simulink model "RobotPID"  (R2023b)
settings: Solver=ode23t  StartTime=0.0  StopTime=inf  RelTol=1e-3
InitFcn:
  | RPInit
StopFcn:
  | run('OccupancyMap.m');
model workspace (MAT data in the model file):
  mapForSim : object (value not decoded)
  occGrid : robotics.BinaryOccupancyGrid (value not decoded)
values from neighbouring files (symbols this model uses):
  X = X + abs(minX)    [OccupancyMap.m]
  Y = Y + abs(minY)    [OccupancyMap.m]
undefined symbols (not defined in the file or in its folder): FloorSurface, Ref, RobotSurface, Z
libraries: sm_lib x21, RP_Simulator_Components x13, nesl_utility x11, RoboticsPlayground x6, slpidlib x2
(part 2 of 2)

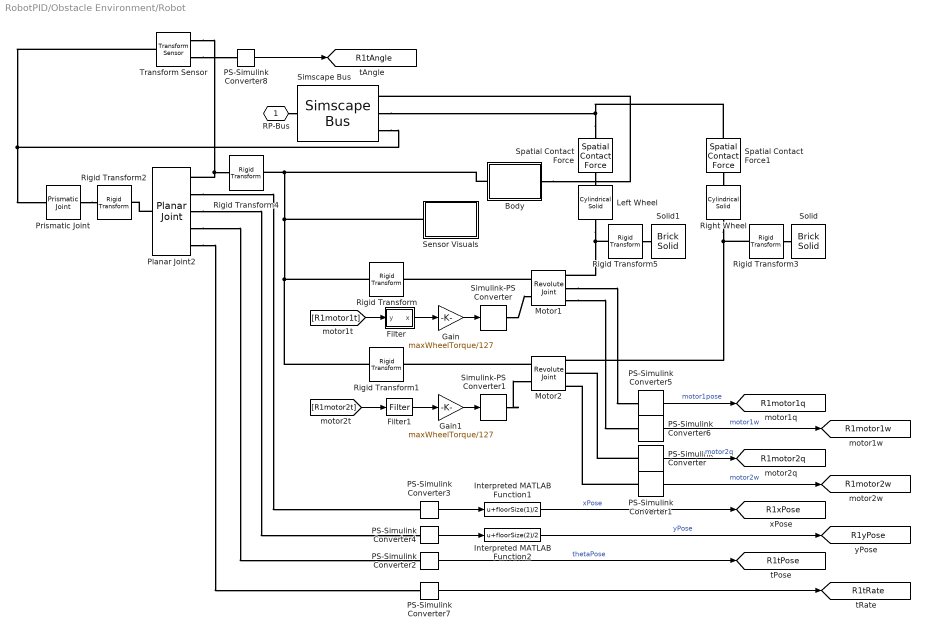
== system RobotPID/Obstacle Environment/Robot ==
  Body : Subsystem
  Filter : Subsystem
  Filter1 : RP_Simulator_Components/Contact Tank Robot/Filter  SystemSampleTime=-1  VariantActivationTime=update diagram  AllowFlexibleInterface=on  Latency=0  AutoFrameSizeCalculation=off
  Gain : Gain  Gain=maxWheelTorque/127
  Gain1 : Gain  Gain=maxWheelTorque/127
  Interpreted MATLAB Function1 : MATLABFcn  MATLABFcn=u+floorSize(1)/2
  Interpreted MATLAB Function2 : MATLABFcn  MATLABFcn=u+floorSize(2)/2
  Left Wheel : sm_lib/Body Elements/Cylindrical Solid  GraphicAmbientColor=[0.15 0.15 0.15 1.0]  BasedOnType=Mass  CenterOfMass=[0 0 0]  CenterOfMassUnits=m  GraphicDiffuseColor=wheelColor  CylinderLength=wheelThickness  CylinderLengthUnits=m  CylinderRadius=wheelRadius  CylinderRadiusUnits=m  Density=1000  DensityUnits=kg/m^3  DoExposeReferenceFrame=on  GraphicEmissiveColor=[0.0 0.0 0.0 1.0]  ExportEntireGeometry=on  SerializedFrames=<Frames/>  MarkerShape=Sphere  MarkerSize=10  GraphicType=FromGeometry  InertiaType=CalculateFromGeometry  Mass=wheelMass  MassUnits=kg  MomentsOfInertia=[1 1 1]  MomentsOfInertiaUnits=kg*m^2  GraphicOpacity=1.0  ProductsOfInertia=[1 1 1]  ProductsOfInertiaUnits=kg*m^2  GraphicShininess=75  GraphicSpecularColor=[0.5 0.5 0.5 1.0]  GraphicVisPropType=SimpleVisualProperties
  Motor1 : sm_lib/Joints/Revolute Joint  JointMode=Normal  SenseConstraintForce=off  SenseConstraintForceX=off  SenseConstraintForceY=off  SenseConstraintForceZ=off  SenseConstraintTorque=off  SenseConstraintTorqueX=off  SenseConstraintTorqueY=off  SenseConstraintTorqueZ=off  SenseTotalForce=off  SenseTotalForceX=off  SenseTotalForceY=off  SenseTotalForceZ=off  SenseTotalTorque=off  SenseTotalTorqueX=off  SenseTotalTorqueY=off  SenseTotalTorqueZ=off  CompositeWrenchDir=FollowerOnBase  CompositeWrenchFrame=BaseFrame  EquilibriumPosition=0  EquilibriumPositionUnits=deg  SpringStiffness=0  SpringStiffnessUnits=N*m/deg  DampingCoefficient=0.004  DampingCoefficientUnits=N*m/(deg/s)  TorqueActuationMode=InputTorque  MotionActuationMode=ComputedMotion  SensePosition=on  SenseVelocity=on  SenseAcceleration=off  SenseTorqueForce=off  SenseLowerLimitTorqueForce=off  SenseUpperLimitTorqueForce=off  LowerLimitSpecify=off  LowerLimitBound=-90  LowerLimitBoundUnits=deg  LowerLimitStiffness=1e4  LowerLimitStiffnessUnits=N*m/deg  LowerLimitDamping=10  LowerLimitDampingUnits=N*m/(deg/s)  LowerLimitTransitionRegionWidth=0.1  LowerLimitTransitionRegionWidthUnits=deg  UpperLimitSpecify=off  UpperLimitBound=90  UpperLimitBoundUnits=deg  UpperLimitStiffness=1e4  UpperLimitStiffnessUnits=N*m/deg  UpperLimitDamping=10  UpperLimitDampingUnits=N*m/(deg/s)  UpperLimitTransitionRegionWidth=0.1  UpperLimitTransitionRegionWidthUnits=deg  PositionTargetSpecify=off  PositionTargetPriority=High  PositionTargetValue=0  PositionTargetValueUnits=deg  VelocityTargetSpecify=off  VelocityTargetPriority=High  VelocityTargetValue=0  VelocityTargetValueUnits=deg/s
  Motor2 : sm_lib/Joints/Revolute Joint  JointMode=Normal  SenseConstraintForce=off  SenseConstraintForceX=off  SenseConstraintForceY=off  SenseConstraintForceZ=off  SenseConstraintTorque=off  SenseConstraintTorqueX=off  SenseConstraintTorqueY=off  SenseConstraintTorqueZ=off  SenseTotalForce=off  SenseTotalForceX=off  SenseTotalForceY=off  SenseTotalForceZ=off  SenseTotalTorque=off  SenseTotalTorqueX=off  SenseTotalTorqueY=off  SenseTotalTorqueZ=off  CompositeWrenchDir=FollowerOnBase  CompositeWrenchFrame=BaseFrame  EquilibriumPosition=0  EquilibriumPositionUnits=deg  SpringStiffness=0  SpringStiffnessUnits=N*m/deg  DampingCoefficient=0.004  DampingCoefficientUnits=N*m/(deg/s)  TorqueActuationMode=InputTorque  MotionActuationMode=ComputedMotion  SensePosition=on  SenseVelocity=on  SenseAcceleration=off  SenseTorqueForce=off  SenseLowerLimitTorqueForce=off  SenseUpperLimitTorqueForce=off  LowerLimitSpecify=off  LowerLimitBound=-90  LowerLimitBoundUnits=deg  LowerLimitStiffness=1e4  LowerLimitStiffnessUnits=N*m/deg  LowerLimitDamping=10  LowerLimitDampingUnits=N*m/(deg/s)  LowerLimitTransitionRegionWidth=0.1  LowerLimitTransitionRegionWidthUnits=deg  UpperLimitSpecify=off  UpperLimitBound=90  UpperLimitBoundUnits=deg  UpperLimitStiffness=1e4  UpperLimitStiffnessUnits=N*m/deg  UpperLimitDamping=10  UpperLimitDampingUnits=N*m/(deg/s)  UpperLimitTransitionRegionWidth=0.1  UpperLimitTransitionRegionWidthUnits=deg  PositionTargetSpecify=off  PositionTargetPriority=High  PositionTargetValue=0  PositionTargetValueUnits=deg  VelocityTargetSpecify=off  VelocityTargetPriority=High  VelocityTargetValue=0  VelocityTargetValueUnits=deg/s
  PS-Simulink Converter{,1,3..6} (6 alike) : nesl_utility/PS-Simulink Converter  PhysicalDomain=network_engine_domain  SubClassName=ps_output  LeftPortType=input  RightPortType=output  PseudoPeriodic=off  Frequencies=[]  VectorFormat=1-D array  Unit=1  AffineConversion=off
  PS-Simulink Converter2 : nesl_utility/PS-Simulink Converter  PhysicalDomain=network_engine_domain  SubClassName=ps_output  LeftPortType=input  RightPortType=output  PseudoPeriodic=off  Frequencies=[]  VectorFormat=1-D array  Unit=rad  AffineConversion=off
  PS-Simulink Converter7 : nesl_utility/PS-Simulink Converter  PhysicalDomain=network_engine_domain  SubClassName=ps_output  LeftPortType=input  RightPortType=output  PseudoPeriodic=off  Frequencies=[]  VectorFormat=1-D array  Unit=deg/s  AffineConversion=off
  PS-Simulink Converter8 : nesl_utility/PS-Simulink Converter  PhysicalDomain=network_engine_domain  SubClassName=ps_output  LeftPortType=input  RightPortType=output  PseudoPeriodic=off  Frequencies=[]  VectorFormat=1-D array  Unit=deg  AffineConversion=off
  Planar Joint2 : sm_lib/Joints/Planar Joint  JointMode=Normal  SenseConstraintForce=off  SenseConstraintForceX=off  SenseConstraintForceY=off  SenseConstraintForceZ=off  SenseConstraintTorque=off  SenseConstraintTorqueX=off  SenseConstraintTorqueY=off  SenseConstraintTorqueZ=off  SenseTotalForce=off  SenseTotalForceX=off  SenseTotalForceY=off  SenseTotalForceZ=off  SenseTotalTorque=off  SenseTotalTorqueX=off  SenseTotalTorqueY=off  SenseTotalTorqueZ=off  CompositeWrenchDir=FollowerOnBase  CompositeWrenchFrame=BaseFrame  PxEquilibriumPosition=0  PxEquilibriumPositionUnits=m  PxSpringStiffness=0  PxSpringStiffnessUnits=N/m  PxDampingCoefficient=5  PxDampingCoefficientUnits=N/(m/s)  PxTorqueActuationMode=NoTorque  PxMotionActuationMode=ComputedMotion  PxSensePosition=on  PxSenseVelocity=off  PxSenseAcceleration=off  PxSenseTorqueForce=off  PxSenseLowerLimitTorqueForce=off  PxSenseUpperLimitTorqueForce=off  PxLowerLimitSpecify=off  PxLowerLimitBound=-1  PxLowerLimitBoundUnits=m  PxLowerLimitStiffness=1e6  PxLowerLimitStiffnessUnits=N/m  PxLowerLimitDamping=1e3  PxLowerLimitDampingUnits=N/(m/s)  PxLowerLimitTransitionRegionWidth=1e-4  PxLowerLimitTransitionRegionWidthUnits=m  PxUpperLimitSpecify=off  PxUpperLimitBound=1  PxUpperLimitBoundUnits=m  PxUpperLimitStiffness=1e6  PxUpperLimitStiffnessUnits=N/m  PxUpperLimitDamping=1e3  PxUpperLimitDampingUnits=N/(m/s)  PxUpperLimitTransitionRegionWidth=1e-4  PxUpperLimitTransitionRegionWidthUnits=m  PxPositionTargetSpecify=on  PxPositionTargetPriority=High  PxPositionTargetValue=startPose(1)  PxPositionTargetValueUnits=m  PxVelocityTargetSpecify=off  PxVelocityTargetPriority=High  PxVelocityTargetValue=0  PxVelocityTargetValueUnits=m/s  PyEquilibriumPosition=0  PyEquilibriumPositionUnits=m  PySpringStiffness=0  PySpringStiffnessUnits=N/m  PyDampingCoefficient=5  PyDampingCoefficientUnits=N/(m/s)  PyTorqueActuationMode=NoTorque  PyMotionActuationMode=ComputedMotion  PySensePosition=on  PySenseVelocity=off  PySenseAcceleration=off  PySenseTorqueForce=off  PySenseLowerLimitTorqueForce=off  PySenseUpperLimitTorqueForce=off  PyLowerLimitSpecify=off  PyLowerLimitBound=-1  PyLowerLimitBoundUnits=m  PyLowerLimitStiffness=1e6  PyLowerLimitStiffnessUnits=N/m  PyLowerLimitDamping=1e3  PyLowerLimitDampingUnits=N/(m/s)  PyLowerLimitTransitionRegionWidth=1e-4  PyLowerLimitTransitionRegionWidthUnits=m  PyUpperLimitSpecify=off  PyUpperLimitBound=1  PyUpperLimitBoundUnits=m  PyUpperLimitStiffness=1e6  PyUpperLimitStiffnessUnits=N/m  PyUpperLimitDamping=1e3  PyUpperLimitDampingUnits=N/(m/s)  PyUpperLimitTransitionRegionWidth=1e-4  PyUpperLimitTransitionRegionWidthUnits=m  PyPositionTargetSpecify=on  PyPositionTargetPriority=High  PyPositionTargetValue=startPose(2)  PyPositionTargetValueUnits=m  PyVelocityTargetSpecify=off  PyVelocityTargetPriority=High  PyVelocityTargetValue=0  PyVelocityTargetValueUnits=m/s  RzEquilibriumPosition=0  RzEquilibriumPositionUnits=deg  RzSpringStiffness=0  RzSpringStiffnessUnits=N*m/deg  RzDampingCoefficient=2/45  RzDampingCoefficientUnits=N*m/(deg/s)  RzTorqueActuationMode=NoTorque  RzMotionActuationMode=ComputedMotion  RzSensePosition=on  RzSenseVelocity=on  RzSenseAcceleration=off  RzSenseTorqueForce=off  RzSenseLowerLimitTorqueForce=off  RzSenseUpperLimitTorqueForce=off  RzLowerLimitSpecify=off  RzLowerLimitBound=-90  RzLowerLimitBoundUnits=deg  RzLowerLimitStiffness=1e4  RzLowerLimitStiffnessUnits=N*m/deg  RzLowerLimitDamping=10  RzLowerLimitDampingUnits=N*m/(deg/s)  RzLowerLimitTransitionRegionWidth=0.1  RzLowerLimitTransitionRegionWidthUnits=deg  RzUpperLimitSpecify=off  RzUpperLimitBound=90  RzUpperLimitBoundUnits=deg  RzUpperLimitStiffness=1e4  RzUpperLimitStiffnessUnits=N*m/deg  RzUpperLimitDamping=10  RzUpperLimitDampingUnits=N*m/(deg/s)  RzUpperLimitTransitionRegionWidth=0.1  RzUpperLimitTransitionRegionWidthUnits=deg  RzPositionTargetSpecify=off  RzPositionTargetPriority=High  RzPositionTargetValue=0  RzPositionTargetValueUnits=deg  RzVelocityTargetSpecify=off  RzVelocityTargetPriority=High  RzVelocityTargetValue=0  RzVelocityTargetValueUnits=deg/s
  Prismatic Joint : sm_lib/Joints/Prismatic Joint  JointMode=Normal  SenseConstraintForce=off  SenseConstraintForceX=off  SenseConstraintForceY=off  SenseConstraintForceZ=off  SenseConstraintTorque=off  SenseConstraintTorqueX=off  SenseConstraintTorqueY=off  SenseConstraintTorqueZ=off  SenseTotalForce=off  SenseTotalForceX=off  SenseTotalForceY=off  SenseTotalForceZ=off  SenseTotalTorque=off  SenseTotalTorqueX=off  SenseTotalTorqueY=off  SenseTotalTorqueZ=off  CompositeWrenchDir=FollowerOnBase  CompositeWrenchFrame=BaseFrame  EquilibriumPosition=0  EquilibriumPositionUnits=m  SpringStiffness=0  SpringStiffnessUnits=N/m  DampingCoefficient=0  DampingCoefficientUnits=N/(m/s)  TorqueActuationMode=NoTorque  MotionActuationMode=ComputedMotion  SensePosition=off  SenseVelocity=off  SenseAcceleration=off  SenseTorqueForce=off  SenseLowerLimitTorqueForce=off  SenseUpperLimitTorqueForce=off  LowerLimitSpecify=off  LowerLimitBound=-1  LowerLimitBoundUnits=m  LowerLimitStiffness=1e6  LowerLimitStiffnessUnits=N/m  LowerLimitDamping=1e3  LowerLimitDampingUnits=N/(m/s)  LowerLimitTransitionRegionWidth=1e-4  LowerLimitTransitionRegionWidthUnits=m  UpperLimitSpecify=off  UpperLimitBound=1  UpperLimitBoundUnits=m  UpperLimitStiffness=1e6  UpperLimitStiffnessUnits=N/m  UpperLimitDamping=1e3  UpperLimitDampingUnits=N/(m/s)  UpperLimitTransitionRegionWidth=1e-4  UpperLimitTransitionRegionWidthUnits=m  PositionTargetSpecify=on  PositionTargetPriority=High  PositionTargetValue=0.02  PositionTargetValueUnits=m  VelocityTargetSpecify=off  VelocityTargetPriority=High  VelocityTargetValue=0  VelocityTargetValueUnits=m/s
  Right Wheel : sm_lib/Body Elements/Cylindrical Solid  GraphicAmbientColor=[0.15 0.15 0.15 1.0]  BasedOnType=Mass  CenterOfMass=[0 0 0]  CenterOfMassUnits=m  GraphicDiffuseColor=wheelColor  CylinderLength=wheelThickness  CylinderLengthUnits=m  CylinderRadius=wheelRadius  CylinderRadiusUnits=m  Density=1000  DensityUnits=kg/m^3  DoExposeReferenceFrame=on  GraphicEmissiveColor=[0.0 0.0 0.0 1.0]  ExportEntireGeometry=on  SerializedFrames=<Frames/>  MarkerShape=Sphere  MarkerSize=10  GraphicType=FromGeometry  InertiaType=CalculateFromGeometry  Mass=wheelMass  MassUnits=kg  MomentsOfInertia=[1 1 1]  MomentsOfInertiaUnits=kg*m^2  GraphicOpacity=1.0  ProductsOfInertia=[1 1 1]  ProductsOfInertiaUnits=kg*m^2  GraphicShininess=75  GraphicSpecularColor=[0.5 0.5 0.5 1.0]  GraphicVisPropType=SimpleVisualProperties
  Rigid Transform : sm_lib/Frames and Transforms/Rigid Transform  TranslationMethod=StandardAxis  TranslationStandardOffset=wheelBase/2  TranslationStandardOffsetUnits=m  TranslationStandardAxis=+Y  TranslationCartesianOffset=[0 0 0]  TranslationCartesianOffsetUnits=m  TranslationROffset=0  TranslationROffsetUnits=m  TranslationZOffset=0  TranslationZOffsetUnits=m  TranslationThetaOffset=0  TranslationThetaOffsetUnits=deg  RotationMethod=AlignedAxes  RotationAngleUnits=deg  RotationStandardAxis=+Z  RotationAngle=0.0  RotationArbitraryAxis=[0 0 1]  FollAlignAxisA=+Z  BaseAlignAxisA=+Y  FollAlignAxisB=+X  BaseAlignAxisB=+X  RotationSequenceAxes=FollowerAxes  RotationSequence=XYX  RotationSequenceAngles=[0 0 0]  RotationSequenceAnglesUnits=deg  RotationMatrix=[1 0 0; 0 1 0; 0 0 1]  Quaternion=[1 0 0 0]
  Rigid Transform1 : sm_lib/Frames and Transforms/Rigid Transform  TranslationMethod=StandardAxis  TranslationStandardOffset=wheelBase/2  TranslationStandardOffsetUnits=m  TranslationStandardAxis=-Y  TranslationCartesianOffset=[0 0 0]  TranslationCartesianOffsetUnits=m  TranslationROffset=0  TranslationROffsetUnits=m  TranslationZOffset=0  TranslationZOffsetUnits=m  TranslationThetaOffset=0  TranslationThetaOffsetUnits=deg  RotationMethod=AlignedAxes  RotationAngleUnits=deg  RotationStandardAxis=+Z  RotationAngle=0.0  RotationArbitraryAxis=[0 0 1]  FollAlignAxisA=+Z  BaseAlignAxisA=+Y  FollAlignAxisB=+X  BaseAlignAxisB=+X  RotationSequenceAxes=FollowerAxes  RotationSequence=XYX  RotationSequenceAngles=[0 0 0]  RotationSequenceAnglesUnits=deg  RotationMatrix=[1 0 0; 0 1 0; 0 0 1]  Quaternion=[1 0 0 0]
  Rigid Transform2 : sm_lib/Frames and Transforms/Rigid Transform  TranslationMethod=StandardAxis  TranslationStandardOffset=wheelRadius  TranslationStandardOffsetUnits=m  TranslationStandardAxis=+Z  TranslationCartesianOffset=[0 0 0]  TranslationCartesianOffsetUnits=m  TranslationROffset=0  TranslationROffsetUnits=m  TranslationZOffset=0  TranslationZOffsetUnits=m  TranslationThetaOffset=0  TranslationThetaOffsetUnits=deg  RotationMethod=None  RotationAngleUnits=deg  RotationStandardAxis=+Z  RotationAngle=0.0  RotationArbitraryAxis=[0 0 1]  FollAlignAxisA=+Z  BaseAlignAxisA=+Y  FollAlignAxisB=+X  BaseAlignAxisB=+X  RotationSequenceAxes=FollowerAxes  RotationSequence=XYX  RotationSequenceAngles=[0 0 0]  RotationSequenceAnglesUnits=deg  RotationMatrix=[1 0 0; 0 1 0; 0 0 1]  Quaternion=[1 0 0 0]
  Rigid Transform3 : sm_lib/Frames and Transforms/Rigid Transform  TranslationMethod=Cartesian  TranslationStandardOffset=0  TranslationStandardOffsetUnits=m  TranslationStandardAxis=+Z  TranslationCartesianOffset=[wheelRadius/2 0 0]  TranslationCartesianOffsetUnits=m  TranslationROffset=0  TranslationROffsetUnits=m  TranslationZOffset=0  TranslationZOffsetUnits=m  TranslationThetaOffset=0  TranslationThetaOffsetUnits=deg  RotationMethod=None  RotationAngleUnits=deg  RotationStandardAxis=+Z  RotationAngle=0.0  RotationArbitraryAxis=[0 0 1]  FollAlignAxisA=+X  BaseAlignAxisA=+Y  FollAlignAxisB=+Y  BaseAlignAxisB=+Z  RotationSequenceAxes=FollowerAxes  RotationSequence=XYX  RotationSequenceAngles=[0 0 0]  RotationSequenceAnglesUnits=deg  RotationMatrix=[1 0 0; 0 1 0; 0 0 1]  Quaternion=[1 0 0 0]
  Rigid Transform4 : sm_lib/Frames and Transforms/Rigid Transform  TranslationMethod=None  TranslationStandardOffset=0  TranslationStandardOffsetUnits=m  TranslationStandardAxis=+Z  TranslationCartesianOffset=[0 0 0]  TranslationCartesianOffsetUnits=m  TranslationROffset=0  TranslationROffsetUnits=m  TranslationZOffset=0  TranslationZOffsetUnits=m  TranslationThetaOffset=0  TranslationThetaOffsetUnits=deg  RotationMethod=StandardAxis  RotationAngleUnits=deg  RotationStandardAxis=+Z  RotationAngle=180*choice  RotationArbitraryAxis=[0 0 1]  FollAlignAxisA=+X  BaseAlignAxisA=+Y  FollAlignAxisB=+Y  BaseAlignAxisB=+Z  RotationSequenceAxes=FollowerAxes  RotationSequence=XYX  RotationSequenceAngles=[0 0 0]  RotationSequenceAnglesUnits=deg  RotationMatrix=[1 0 0; 0 1 0; 0 0 1]  Quaternion=[1 0 0 0]
  Rigid Transform5 : sm_lib/Frames and Transforms/Rigid Transform  TranslationMethod=Cartesian  TranslationStandardOffset=0  TranslationStandardOffsetUnits=m  TranslationStandardAxis=+Z  TranslationCartesianOffset=[wheelRadius/2 0 0]  TranslationCartesianOffsetUnits=m  TranslationROffset=0  TranslationROffsetUnits=m  TranslationZOffset=0  TranslationZOffsetUnits=m  TranslationThetaOffset=0  TranslationThetaOffsetUnits=deg  RotationMethod=None  RotationAngleUnits=deg  RotationStandardAxis=+Z  RotationAngle=0.0  RotationArbitraryAxis=[0 0 1]  FollAlignAxisA=+X  BaseAlignAxisA=+Y  FollAlignAxisB=+Y  BaseAlignAxisB=+Z  RotationSequenceAxes=FollowerAxes  RotationSequence=XYX  RotationSequenceAngles=[0 0 0]  RotationSequenceAnglesUnits=deg  RotationMatrix=[1 0 0; 0 1 0; 0 0 1]  Quaternion=[1 0 0 0]
  Sensor Visuals : Subsystem
  Simscape Bus : SimscapeBus  HierarchyStrings=RobotSurface;FloorSurface;Ref
  Simulink-PS Converter : nesl_utility/Simulink-PS Converter  PhysicalDomain=network_engine_domain  SubClassName=ps_input  LeftPortType=input  RightPortType=output  PseudoPeriodic=off  Frequencies=[]  NoiseDistribution=none  NoiseParameters=[]  Unit=1  AffineConversion=off  FilteringAndDerivatives=provide  SimscapeFilterOrder=1  InputFilterTimeConstant=0.05  UdotUserProvided=0
  Simulink-PS Converter1 : nesl_utility/Simulink-PS Converter  PhysicalDomain=network_engine_domain  SubClassName=ps_input  LeftPortType=input  RightPortType=output  PseudoPeriodic=off  Frequencies=[]  NoiseDistribution=none  NoiseParameters=[]  Unit=1  AffineConversion=off  FilteringAndDerivatives=provide  SimscapeFilterOrder=1  InputFilterTimeConstant=0.05  UdotUserProvided=0
  Solid : sm_lib/Body Elements/Brick Solid  GraphicAmbientColor=[0.15 0.15 0.15 1.0]  BasedOnType=Density  BrickDimensions=[wheelRadius*0.8 wheelThickness*1.05 wheelThickness*1.05]  BrickDimensionsUnits=m  CenterOfMass=[0 0 0]  CenterOfMassUnits=m  GraphicDiffuseColor=[0.0 0.8 0.8]  Density=1000  DensityUnits=kg/m^3  DoExposeReferenceFrame=on  GraphicEmissiveColor=[0.0 0.0 0.0 1.0]  ExportEntireGeometry=off  SerializedFrames=<Frames/>  MarkerShape=Sphere  MarkerSize=10  GraphicType=FromGeometry  InertiaType=CalculateFromGeometry  Mass=1  MassUnits=kg  MomentsOfInertia=[1 1 1]  MomentsOfInertiaUnits=kg*m^2  GraphicOpacity=1.0  ProductsOfInertia=[1 1 1]  ProductsOfInertiaUnits=kg*m^2  GraphicShininess=75  GraphicSpecularColor=[0.5 0.5 0.5 1.0]  GraphicVisPropType=SimpleVisualProperties
  Solid1 : sm_lib/Body Elements/Brick Solid  GraphicAmbientColor=[0.15 0.15 0.15 1.0]  BasedOnType=Density  BrickDimensions=[wheelRadius*0.8 wheelThickness*1.05 wheelThickness*1.05]  BrickDimensionsUnits=m  CenterOfMass=[0 0 0]  CenterOfMassUnits=m  GraphicDiffuseColor=[0.0 0.8 0.8]  Density=1000  DensityUnits=kg/m^3  DoExposeReferenceFrame=on  GraphicEmissiveColor=[0.0 0.0 0.0 1.0]  ExportEntireGeometry=off  SerializedFrames=<Frames/>  MarkerShape=Sphere  MarkerSize=10  GraphicType=FromGeometry  InertiaType=CalculateFromGeometry  Mass=1  MassUnits=kg  MomentsOfInertia=[1 1 1]  MomentsOfInertiaUnits=kg*m^2  GraphicOpacity=1.0  ProductsOfInertia=[1 1 1]  ProductsOfInertiaUnits=kg*m^2  GraphicShininess=75  GraphicSpecularColor=[0.5 0.5 0.5 1.0]  GraphicVisPropType=SimpleVisualProperties
  Spatial Contact Force : sm_lib/Forces and Torques/Spatial Contact Force  SenseContactBaseRotation=off  SenseContactBaseTranslation=off  CoefficientOfDynamicFriction=0.5  CoefficientOfStaticFriction=0.7  NormalDamping=1e2  NormalDampingUnits=N/(m/s)  SenseContactSignal=off  NormalStiffness=1e4  NormalStiffnessUnits=N/m  FrictionalCriticalVelocity=1e-3  FrictionalCriticalVelocityUnits=m/s  ZeroCrossDetectContactStartAndEnd=off  SenseContactFollowerRotation=off  SenseContactFollowerTranslation=off  FrictionType=SmoothStickSlip  SenseFrictionalForceMagnitude=off  SenseNormalForceMagnitude=off  NormalForceType=SmoothSpringDamper  SenseNormalVelocity=off  SensePenetrationDepth=off  SenseSeparationDistance=off  SenseTangentialVelocity=off  NormalTransitionRegionWidth=1e-4  NormalTransitionRegionWidthUnits=m
  Spatial Contact Force1 : sm_lib/Forces and Torques/Spatial Contact Force  SenseContactBaseRotation=off  SenseContactBaseTranslation=off  CoefficientOfDynamicFriction=0.5  CoefficientOfStaticFriction=0.7  NormalDamping=1e2  NormalDampingUnits=N/(m/s)  SenseContactSignal=off  NormalStiffness=1e4  NormalStiffnessUnits=N/m  FrictionalCriticalVelocity=1e-3  FrictionalCriticalVelocityUnits=m/s  ZeroCrossDetectContactStartAndEnd=off  SenseContactFollowerRotation=off  SenseContactFollowerTranslation=off  FrictionType=SmoothStickSlip  SenseFrictionalForceMagnitude=off  SenseNormalForceMagnitude=off  NormalForceType=SmoothSpringDamper  SenseNormalVelocity=off  SensePenetrationDepth=off  SenseSeparationDistance=off  SenseTangentialVelocity=off  NormalTransitionRegionWidth=1e-4  NormalTransitionRegionWidthUnits=m
  Transform Sensor : sm_lib/Frames and Transforms/Transform Sensor  MeasurementFrame=World  RotationSequence=XYX  SenseAngle=on  SenseAxis=off  SenseQ=off  SenseR=off  SenseRotationSequence=off  SenseOmegaX=off  SenseOmegaY=off  SenseOmegaZ=off  SenseOmega=off  SenseQDot=off  SenseRDot=off  SenseRotationSequenceDot=off  SenseAlphaX=off  SenseAlphaY=off  SenseAlphaZ=off  SenseAlpha=off  SenseQDDot=off  SenseRDDot=off  SenseX=off  SenseY=off  SenseZ=off  SenseXYZ=off  SenseRad=off  SenseAzim=off  SenseDist=off  SenseInc=off  SenseXDot=off  SenseYDot=off  SenseZDot=off  SenseXYZDot=off  SenseRadDot=off  SenseAzimDot=off  SenseDistDot=off  SenseIncDot=off  SenseXDDot=off  SenseYDDot=off  SenseZDDot=off  SenseXYZDDot=off  SenseRadDDot=off  SenseAzimDDot=off  SenseDistDDot=off  SenseIncDDot=off
  RP-Bus : PMIOPort  Side=Right
  tag scope: R1motor1q=global, R1motor1w=global, R1motor2q=global, R1motor2w=global, R1tAngle=global, R1tPose=global, R1tRate=global, R1xPose=global, R1yPose=global
  wires:
  PS-Simulink Converter8/1 -> [R1tAngle]
  PS-Simulink Converter7/1 -> [R1tRate]
  PS-Simulink Converter6/1 -> [R1motor1w]  "motor1w"
  PS-Simulink Converter5/1 -> [R1motor1q]  "motor1pose"
  PS-Simulink Converter/1 -> [R1motor2q]  "motor2q"
  PS-Simulink Converter1/1 -> [R1motor2w]  "motor2w"
  Interpreted MATLAB Function2/1 -> [R1yPose]  "yPose"
  Interpreted MATLAB Function1/1 -> [R1xPose]  "xPose"
  PS-Simulink Converter2/1 -> [R1tPose]  "thetaPose"
  PS-Simulink Converter3/1 -> Interpreted MATLAB Function1/1
  PS-Simulink Converter4/1 -> Interpreted MATLAB Function2/1
  Filter1/1 -> Gain1/1
  Filter/1(x) -> Gain/1
  Gain/1 -> Simulink-PS Converter/1
  Gain1/1 -> Simulink-PS Converter1/1
  [R1motor1t] -> Filter/1(y)
  [R1motor2t] -> Filter1/1
  connections:
  Body/RConn1 -- Simscape Bus/LConn1
  Spatial Contact Force1/RConn1 -- Right Wheel/LConn1
  Spatial Contact Force/LConn1 -- Spatial Contact Force1/LConn1 -- Simscape Bus/LConn2
  Spatial Contact Force/RConn1 -- Left Wheel/LConn1
  RP-Bus/RConn1 -- Simscape Bus/RConn1
  Transform Sensor/RConn2 -- PS-Simulink Converter8/LConn1
  Planar Joint2/RConn5 -- PS-Simulink Converter7/LConn1
  Rigid Transform5/RConn1 -- Solid1/RConn1
  Rigid Transform3/RConn1 -- Solid/RConn1
  PS-Simulink Converter1/LConn1 -- Motor2/RConn3
  PS-Simulink Converter/LConn1 -- Motor2/RConn2
  Motor1/RConn3 -- PS-Simulink Converter6/LConn1
  Motor1/RConn2 -- PS-Simulink Converter5/LConn1
  Planar Joint2/RConn4 -- PS-Simulink Converter2/LConn1
  Planar Joint2/RConn3 -- PS-Simulink Converter4/LConn1
  Planar Joint2/RConn2 -- PS-Simulink Converter3/LConn1
  Simulink-PS Converter/RConn1 -- Motor1/LConn2
  Simulink-PS Converter1/RConn1 -- Motor2/LConn2
  Motor2/RConn1 -- Right Wheel/RConn1 -- Rigid Transform3/LConn1
  Motor1/LConn1 -- Rigid Transform/RConn1
  Planar Joint2/LConn1 -- Rigid Transform2/RConn1
  Simscape Bus/LConn3 -- Prismatic Joint/LConn1 -- Transform Sensor/LConn1
  Motor2/LConn1 -- Rigid Transform1/RConn1
  Motor1/RConn1 -- Rigid Transform5/LConn1 -- Left Wheel/RConn1
  Rigid Transform4/RConn1 -- Body/LConn1 -- Sensor Visuals/LConn1 -- Rigid Transform/LConn1 -- Rigid Transform1/LConn1
  Planar Joint2/RConn1 -- Rigid Transform4/LConn1 -- Transform Sensor/RConn1
  Prismatic Joint/RConn1 -- Rigid Transform2/LConn1

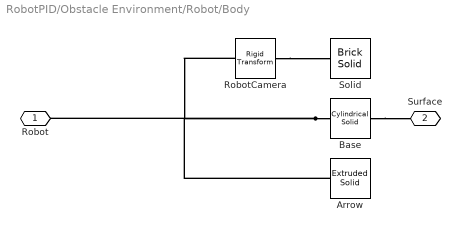
== system RobotPID/Obstacle Environment/Robot/Body ==
  Arrow : sm_lib/Body Elements/Extruded Solid  GraphicAmbientColor=[0.15 0.15 0.15 1.0]  BasedOnType=Density  CenterOfMass=[0 0 0]  CenterOfMassUnits=m  GraphicDiffuseColor=[0.8 0.0 1.0]  ExportConvexHullGeometry=off  ExtrusionCrossSection=[1 1; -1 1; -1 -1; 1 -1]  ExtrusionCrossSectionUnits=m  Density=1000  DensityUnits=kg/m^3  DoExposeReferenceFrame=on  GraphicEmissiveColor=[0.0 0.0 0.0 1.0]  ExportEntireGeometry=off  ExtrusionLength=1.3*chassisThickness  ExtrusionLengthUnits=m  ExtrusionType=Regular  SerializedFrames=<Frames/>  MarkerShape=Sphere  MarkerSize=10  GraphicType=FromGeometry  InertiaType=PointMass  Mass=0.2  MassUnits=kg  MomentsOfInertia=[1 1 1]  MomentsOfInertiaUnits=kg*m^2  PolygonNumSides=3  GraphicOpacity=1.0  PolygonOuterRadius=wheelBase/2-wheelBase*0.15  PolygonOuterRadiusUnits=m  ProductsOfInertia=[1 1 1]  ProductsOfInertiaUnits=kg*m^2  GraphicShininess=75  GraphicSpecularColor=[0.5 0.5 0.5 1.0]  GraphicVisPropType=SimpleVisualProperties
  Base : sm_lib/Body Elements/Cylindrical Solid  GraphicAmbientColor=[0.15 0.15 0.15 1.0]  BasedOnType=Mass  CenterOfMass=[0 0 0]  CenterOfMassUnits=m  GraphicDiffuseColor=chassisColor  CylinderLength=chassisThickness  CylinderLengthUnits=m  CylinderRadius=(wheelBase-wheelThickness)/2  CylinderRadiusUnits=m  Density=chassisMass  DensityUnits=kg/m^3  DoExposeReferenceFrame=on  GraphicEmissiveColor=[0.0 0.0 0.0 1.0]  ExportEntireGeometry=on  SerializedFrames=<Frames/>  MarkerShape=Sphere  MarkerSize=10  GraphicType=FromGeometry  InertiaType=CalculateFromGeometry  Mass=chassisMass  MassUnits=kg  MomentsOfInertia=[1 1 1]  MomentsOfInertiaUnits=kg*m^2  GraphicOpacity=1.0  ProductsOfInertia=[1 1 1]  ProductsOfInertiaUnits=kg*m^2  GraphicShininess=75  GraphicSpecularColor=[0.5 0.5 0.5 1.0]  GraphicVisPropType=SimpleVisualProperties
  RobotCamera : sm_lib/Frames and Transforms/Rigid Transform  TranslationMethod=Cartesian  TranslationStandardOffset=0  TranslationStandardOffsetUnits=m  TranslationStandardAxis=+Z  TranslationCartesianOffset=[-0.5 0 0.35]  TranslationCartesianOffsetUnits=m  TranslationROffset=0  TranslationROffsetUnits=m  TranslationZOffset=0  TranslationZOffsetUnits=m  TranslationThetaOffset=0  TranslationThetaOffsetUnits=deg  RotationMethod=StandardAxis  RotationAngleUnits=deg  RotationStandardAxis=+Y  RotationAngle=20  RotationArbitraryAxis=[0 0 1]  FollAlignAxisA=+X  BaseAlignAxisA=+Y  FollAlignAxisB=+Y  BaseAlignAxisB=+Z  RotationSequenceAxes=FollowerAxes  RotationSequence=XYX  RotationSequenceAngles=[0 0 0]  RotationSequenceAnglesUnits=deg  RotationMatrix=[1 0 0; 0 1 0; 0 0 1]  Quaternion=[1 0 0 0]
  Solid : sm_lib/Body Elements/Brick Solid  GraphicAmbientColor=[0.15 0.15 0.15 1.0]  BasedOnType=Density  BrickDimensions=[0.001 0.001 0.001]  BrickDimensionsUnits=m  CenterOfMass=[0 0 0]  CenterOfMassUnits=m  GraphicDiffuseColor=[0.5 0.5 0.5]  Density=1000  DensityUnits=kg/m^3  DoExposeReferenceFrame=on  GraphicEmissiveColor=[0.0 0.0 0.0 1.0]  ExportEntireGeometry=off  SerializedFrames=<Frames/>  MarkerShape=Sphere  MarkerSize=10  GraphicType=FromGeometry  InertiaType=PointMass  Mass=0.00001  MassUnits=kg  MomentsOfInertia=[1 1 1]  MomentsOfInertiaUnits=kg*m^2  GraphicOpacity=0  ProductsOfInertia=[1 1 1]  ProductsOfInertiaUnits=kg*m^2  GraphicShininess=75  GraphicSpecularColor=[0.5 0.5 0.5 1.0]  GraphicVisPropType=SimpleVisualProperties
  Robot : PMIOPort  Side=Left
  Surface : PMIOPort  Port=2  Side=Right
  connections:
  Base/LConn1 -- Surface/RConn1
  Base/RConn1 -- RobotCamera/LConn1 -- Robot/RConn1 -- Arrow/RConn1
  RobotCamera/RConn1 -- Solid/RConn1

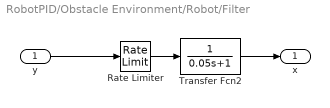
== system RobotPID/Obstacle Environment/Robot/Filter ==
  y : Inport
  Rate Limiter : RateLimiter  RisingSlewLimit=300  FallingSlewLimit=-300  SampleTimeMode=inherited
  Transfer Fcn2 : TransferFcn  Denominator=[0.05 1]
  x : Outport  VectorParamsAs1DForOutWhenUnconnected=off
  wires:
  y/1 -> Rate Limiter/1
  Transfer Fcn2/1 -> x/1
  Rate Limiter/1 -> Transfer Fcn2/1

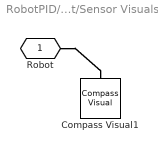
== system RobotPID/Obstacle Environment/Robot/Sensor Visuals ==
  Compass Visual1 : RP_Simulator_Components/Compass Visual  size=0.8  color=[0.1 0.1 0.1]  pose=[0 0]  angle=0
  Robot : PMIOPort  Side=Left
  connections:
  Robot/RConn1 -- Compass Visual1/LConn1

== stateflow chart RobotPID/Robot Controller ==
  state PathPlanning [parallel]
    settings: executionOrder=3
    state getnextmove
      entry:
      map=updateMap(map,F,L01,L04,R12,R15,orientation,position,cell,toll);
      newMoves = callBFS(map,position,orientation);
      if (~isempty(newMoves))
      moves=[moves, newMoves(1)];
      end
      map(position(1),position(2))=2;
      i=i+1;
      goalticks = front_0;
      ahead=0;
      nextmove=moves(i);
    state init
      entry:
      i=0;
      nextmove2=0;
      nextmove=0;
      moves2=[0 0];
      newMoves = [0 0];
      map2=zeros(20,20);
      moves=[0 0];
      map=zeros(20,20);
      position=[10 10];
      map(position(1),position(2))=2;
    state lookahead
      entry:
      map2=updateMap(map,F,L01,L04,R12,R15,orientation,position,cell,toll);
      moves2=callBFS(map2,position,orientation);
      nextmove2=moves2(1);
    state moveforward
      entry:
      goalticks = goalticks + cellsize;
      switch orientation
      case 0
      position(2)=position(2)+1;
      case 90
      position(1)=position(1)-1;
      case 180
      position(2)=position(2)-1;
      case 270
      position(1)=position(1)+1;
      end
      map(position(1),position(2))=2;
    state stillforward
      entry:
      ahead=ahead+1;
      map=map2;
      moves=[moves, nextmove2];
      nextmove=nextmove2;
      i=i+1;
    getnextmove -> getnextmove [order 3] : [nextmove==0]
    lookahead -> getnextmove [order 2] : [(nextmove2~=1) && (in(Navigation.Stop))]{moves=[moves, nextmove2];}
    moveforward -> lookahead : after(0.5,sec)[front - front_0 >= ((cellsize*0.8) + (ahead*cellsize))]
    lookahead -> stillforward [order 1] : [nextmove2==1]
    init -> getnextmove
    getnextmove -> getnextmove [order 2] : after(1,sec)[(nextmove==2 || nextmove==3)&&(in(Navigation.Stop))]
    getnextmove -> moveforward [order 1] : [nextmove==1]
    (default) -> init
    stillforward -> moveforward
  state Orientation [parallel]
    settings: executionOrder=1
    state NORD
      orientation = 90;
    state OVEST
      orientation = 180;
    state EST
      orientation = 0;
    state SUD
      orientation = 270;
    EST -> NORD [order 1] : [in(Navigation.TurnLeft) && compass > 45]
    NORD -> OVEST [order 1] : [in(Navigation.TurnLeft) && compass > 135]
    OVEST -> NORD [order 2] : [in(Navigation.TurnRight) && compass < 135]
    NORD -> EST [order 2] : [in(Navigation.TurnRight) && compass < 45]
    (default) -> EST
    OVEST -> SUD [order 1] : [in(Navigation.TurnLeft) && compass < 135]
    SUD -> OVEST [order 2] : [in(Navigation.TurnRight) && compass > 135]
    SUD -> EST [order 1] : [in(Navigation.TurnLeft) && compass < 45]
    EST -> SUD [order 2] : [in(Navigation.TurnRight) && compass > 45]
  state Navigation [parallel]
    settings: executionOrder=2
    state idle
      entry:
      %end=5,forward=1
      %left=2,right=3
      front_0 = ticks;
      isMoving = 0;
      isRotating = 0;
      front=0;
      degrees=0;
      DONE = 0;
    state forward
      entry:
      isMoving = 1;
      during:
      front = ticks;
    state Stop
      entry:
      isMoving = 0;
      isRotating = 0;
      front_0 = ticks;
    state TurnRight
      entry:
      isRotating = 1;
      degrees=degrees-90;
    state TurnLeft
      entry:
      isRotating = 1;
      degrees=degrees+90;
    (default) -> idle
    Stop -> forward [order 3] : [nextmove==1]
    forward -> Stop : [(goalticks - front) == 0]
    idle -> Stop
    TurnRight -> Stop : after(0.5,sec)[((compass > 89.9 && compass < 90.1) || compass > 179.9 || compass < 0.1)]
    TurnLeft -> Stop : after(0.5,sec)[((compass > 89.9 && compass < 90.1) || compass > 179.9 || compass < 0.1)]
    Stop -> TurnLeft [order 1] : after(0.5,sec)[nextmove==2]
    Stop -> TurnRight [order 2] : after(0.5,sec)[nextmove==3]
    Stop -> Stop [order 4] : after(2,sec)[nextmove==5]{DONE=1}
  data: grid function_input; startPos function_input; startOrientation function_input; path function_output; map function_input; F function_input; L01 function_input; map function_output; L04 function_input; R12 function_input; R15 function_input; o function_input; p function_input; c function_input; t function_input; compass input; orientation output double; front output double; front_0 output double; isMoving output; ticks input; cellsize input; moves local; nextmove local; i local; position local; R12 input; L04 input; F input; toll input; cell input; degrees output; goalticks output; isRotating output; DONE output; moves2 local; map2 local; ahead local; nextmove2 local; newMoves local; L01 input; R15 input; map output
  function path = callBFS(grid, startPos, startOrientation):
    | function path = callBFS(grid, startPos, startOrientation)
    |     coder.extrinsic('bfs_find_closest')
    |     path = bfs_find_closest(grid, startPos, startOrientation);
    | end
  function map=updateMap(map,F,L01,L04,R12,R15,o,p,c,t):
    | function map=updateMap(map,F,L01,L04,R12,R15,o,p,c,t)
    |     coder.extrinsic('mapUpdate')
    |     map = mapUpdate(map,F,L01,L04,R12,R15,o,p,c,t);
    | end

== matlab function RobotPID/MATLAB Function ==
  data: matrixMap input
function showMatrix(matrixMap)
imagesc(matrixMap)

== stateflow chart RobotPID/RobotPose & ObstaclesMapping/PoseMapping ==
  state Case90
    during:
    distanza = ((CurrTicks - temp) * DistTicks)*0.01;
    Y_out = Y_out + distanza;
    O_f = [X_out , Y_out + f];
    O_l01 = [X_out - l01*sin(1*(pi/8)) , Y_out + l01*cos(1*(pi/8))];
    O_l02 = [X_out - l02/sqrt(2) , Y_out + l02/sqrt(2)];
    O_l03 = [X_out - l03*sin(3*(pi/8)) , Y_out + l03*cos(3*(pi/8))];
    O_r01 = [X_out + r01*sin(1*(pi/8)) , Y_out + r01*cos(1*(pi/8))];
    O_r02 = [X_out + r02/sqrt(2) , Y_out + r02/sqrt(2)];
    O_r03 = [X_out + r03*sin(3*(pi/8)) , Y_out + r03*cos(3*(pi/8))];
    temp = CurrTicks;
  state Init
    entry:
    X_out = 0;
    Y_out = 0;
  state Case180
    during:
    distanza = ((CurrTicks - temp) * DistTicks)*0.01;
    X_out = X_out - distanza;
    O_f = [X_out - f , Y_out];
    O_l01 = [X_out - l01*cos(1*(pi/8)) , Y_out - l01*sin(1*(pi/8))];
    O_l02 = [X_out - l02/sqrt(2) , Y_out - l02/sqrt(2)];
    O_l03 = [X_out - l03*cos(3*(pi/8)) , Y_out - l03*sin(3*(pi/8))];
    O_r01 = [X_out - r01*cos(1*(pi/8)) , Y_out + r01*sin(1*(pi/8))];
    O_r02 = [X_out - r02/sqrt(2) , Y_out + r02/sqrt(2)];
    O_r03 = [X_out - r03*cos(3*(pi/8)) , Y_out + r03*sin(3*(pi/8))];
    temp = CurrTicks;
  state Case0
    during:
    distanza = ((CurrTicks - temp) * DistTicks)*0.01;
    X_out = X_out + distanza;
    O_f = [X_out + f , Y_out];
    O_l01 = [X_out + l01*cos(1*(pi/8)) , Y_out + l01*sin(1*(pi/8))];
    O_l02 = [X_out + l02/sqrt(2) , Y_out + l02/sqrt(2)];
    O_l03 = [X_out + l03*cos(3*(pi/8)) , Y_out + l03*sin(3*(pi/8))];
    O_r01 = [X_out + r01*cos(1*(pi/8)) , Y_out - r01*sin(1*(pi/8))];
    O_r02 = [X_out + r02/sqrt(2) , Y_out - r02/sqrt(2)];
    O_r03 = [X_out + r03*cos(3*(pi/8)) , Y_out - r03*sin(3*(pi/8))];
    temp = CurrTicks;
  state Stop
    entry:
    distanza = 0;
    temp = 0;
  state Case270
    during:
    distanza = ((CurrTicks - temp) * DistTicks)*0.01;
    Y_out = Y_out - distanza;
    O_f = [X_out , Y_out - f];
    O_l01 = [X_out + l01*sin(1*(pi/8)) , Y_out - l01*cos(1*(pi/8))];
    O_l02 = [X_out + l02/sqrt(2) , Y_out - l02/sqrt(2)];
    O_l03 = [X_out + l03*sin(3*(pi/8)) , Y_out - l03*cos(3*(pi/8))];
    O_r01 = [X_out - r01*sin(1*(pi/8)) , Y_out - r01*cos(1*(pi/8))];
    O_r02 = [X_out - r02/sqrt(2) , Y_out - r02/sqrt(2)];
    O_r03 = [X_out - r03*sin(3*(pi/8)) , Y_out - r03*cos(3*(pi/8))];
    temp = CurrTicks;
  (default) -> Init
  Init -> Stop
  Stop -> Case90 [order 1] : [IsMoving == 1 && Orientation == 90]{temp = StartTicks;}
  Case90 -> Stop : [IsMoving == 0]
  Case180 -> Stop : [IsMoving == 0]
  Case0 -> Stop : [IsMoving == 0]
  Stop -> Case180 [order 4] : [IsMoving == 1 && Orientation == 180]{temp = StartTicks;}
  Stop -> Case0 [order 2] : [IsMoving == 1 && Orientation == 0]{temp = StartTicks;}
  Stop -> Case270 [order 3] : [IsMoving == 1 && Orientation == 270]{temp = StartTicks;}
  Case270 -> Stop : [IsMoving == 0]
  data: IsMoving input; X_out output; Y_out output; Orientation input; CurrTicks input; StartTicks input; DistTicks input; distanza local; temp local; O_l01 output size=[1 2]; O_l02 output size=[1 2]; O_l03 output size=[1 2]; O_r03 output size=[1 2]; O_r02 output size=[1 2]; O_r01 output size=[1 2]; l01 input; l02 input; l03 input; r03 input; r02 input; r01 input; f input; O_f output size=[1 2]
